simulink model "connections"  (R2020a)
settings: Solver=FixedStepAuto  StartTime=0.0  StopTime=5000  FixedStep=0.1  RelTol=1e-3
values from neighbouring files (symbols this model uses):
  east_drift_limit = 2    [wave_parameters.mat]
  k_down = 1.3    [wave_parameters.mat]
  k_east = 2    [wave_parameters.mat]
  k_north = 2    [wave_parameters.mat]
  k_pitch = 3    [wave_parameters.mat]
  k_roll = 3    [wave_parameters.mat]
  k_yaw = 3    [wave_parameters.mat]
  north_drift_limit = 2    [wave_parameters.mat]
  numberOfBuses = 2    [init.m]
  numberOfGenerators = 4    [init.m]
  peak_frequency = 0.8    [wave_parameters.mat]
  wave_height = 1    [wave_parameters.mat]
  yaw_drift_limit = 0.174532925199    [wave_parameters.mat]
undefined symbols (not defined in the file or in its folder): east, magnitude, north, surge, sway, yaw
libraries: simulink x28, simulink_extras x18
(part 3 of 4)

== system connections/power_plant/Subsystem/Bus array to array1/Bus array to array ==
  In1 : Inport  OutDataTypeStr=Bus: TheveninBus  Partition=on  PartitionDimension=2  PartitionWidth=1  PartitionOffset=0
  Bus Selector : BusSelector  OutputSignals=E,Z,Sb,Connected,omega,SwitchboardID
  For Each : ForEach  DisableCoverage=on
  E : Outport  ConcatenationDimension=2  VectorParamsAs1DForOutWhenUnconnected=off
  Z : Outport  Port=2  ConcatenationDimension=2  VectorParamsAs1DForOutWhenUnconnected=off
  Sb : Outport  Port=3  ConcatenationDimension=2  VectorParamsAs1DForOutWhenUnconnected=off
  Connected : Outport  Port=4  ConcatenationDimension=2  VectorParamsAs1DForOutWhenUnconnected=off
  omega : Outport  Port=5  ConcatenationDimension=2  VectorParamsAs1DForOutWhenUnconnected=off
  SwitchboardID : Outport  Port=6  ConcatenationDimension=2  VectorParamsAs1DForOutWhenUnconnected=off
  wires:
  Bus Selector/6 -> SwitchboardID/1  "<SwitchboardID>"
  Bus Selector/5 -> omega/1  "<omega>"
  Bus Selector/4 -> Connected/1  "<Connected>"
  Bus Selector/3 -> Sb/1  "<Sb>"
  Bus Selector/1 -> E/1  "<E>"
  Bus Selector/2 -> Z/1  "<Z>"
  In1/1 -> Bus Selector/1

== system connections/power_plant/Subsystem/Merger/For Each Subsystem ==
  v : Inport  Partition=on  PartitionDimension=2  PartitionWidth=1  PartitionOffset=0
  omega : Inport  Port=2  Partition=on  PartitionDimension=2  PartitionWidth=1  PartitionOffset=0
  theta : Inport  Port=3  Partition=on  PartitionDimension=2  PartitionWidth=1  PartitionOffset=0
  Bus Creator : BusCreator  Inputs=3  OutDataTypeStr=Bus: swb  NonVirtualBus=on
  For Each : ForEach  DisableCoverage=on
  Out1 : Outport  OutDataTypeStr=Bus: swb  ConcatenationDimension=2  VectorParamsAs1DForOutWhenUnconnected=off
  wires:
  Bus Creator/1 -> Out1/1
  v/1 -> Bus Creator/1  "voltage"
  omega/1 -> Bus Creator/2  "omega"
  theta/1 -> Bus Creator/3  "thetaElectric"

== system connections/power_plant/Subsystem1/Subsystem1/Bus array to array ==
  In1 : Inport  OutDataTypeStr=Bus: TheveninBus  Partition=on  PartitionDimension=1  PartitionWidth=1  PartitionOffset=0
  Bus array to array : Subsystem  TreatAsAtomicUnit=on
  For Each : ForEach  DisableCoverage=on
  E : Outport  ConcatenationDimension=1  VectorParamsAs1DForOutWhenUnconnected=off
  Z : Outport  Port=2  ConcatenationDimension=1  VectorParamsAs1DForOutWhenUnconnected=off
  Sb : Outport  Port=3  ConcatenationDimension=1  VectorParamsAs1DForOutWhenUnconnected=off
  Connected : Outport  Port=4  ConcatenationDimension=1  VectorParamsAs1DForOutWhenUnconnected=off
  omega : Outport  Port=5  ConcatenationDimension=1  VectorParamsAs1DForOutWhenUnconnected=off
  SwitchboardID : Outport  Port=6  ConcatenationDimension=1  VectorParamsAs1DForOutWhenUnconnected=off
  wires:
  Bus array to array/6(SwitchboardID) -> SwitchboardID/1
  Bus array to array/5(omega) -> omega/1
  Bus array to array/4(Connected) -> Connected/1
  Bus array to array/3(Sb) -> Sb/1
  Bus array to array/1(E) -> E/1
  Bus array to array/2(Z) -> Z/1
  In1/1 -> Bus array to array/1(In1)

== system connections/power_plant/Subsystem1/Subsystem1/For Each Subsystem1 ==
  E : Inport  Partition=on  PartitionDimension=1  PartitionWidth=1  PartitionOffset=0
  Z : Inport  Port=2  Partition=on  PartitionDimension=1  PartitionWidth=1  PartitionOffset=0
  Sb : Inport  Port=3  Partition=on  PartitionDimension=1  PartitionWidth=1  PartitionOffset=0
  Connected : Inport  Port=4  Partition=on  PartitionDimension=1  PartitionWidth=1  PartitionOffset=0
  omega : Inport  Port=5  Partition=on  PartitionDimension=1  PartitionWidth=1  PartitionOffset=0
  SwitchboardID : Inport  Port=6  Partition=on  PartitionDimension=1  PartitionWidth=1  PartitionOffset=0
  For Each : ForEach  DisableCoverage=on
  For Each Subsystem : Subsystem  TreatAsAtomicUnit=on
  Out1 : Outport  OutDataTypeStr=Bus: TheveninBus  ConcatenationDimension=1  VectorParamsAs1DForOutWhenUnconnected=off
  wires:
  For Each Subsystem/1(Out1) -> Out1/1
  SwitchboardID/1 -> For Each Subsystem/6(SwitchboardID)  "SwitchboardID"
  omega/1 -> For Each Subsystem/5(omega)  "omega"
  Connected/1 -> For Each Subsystem/4(Connected)  "Connected"
  Sb/1 -> For Each Subsystem/3(Sb)  "Sb"
  Z/1 -> For Each Subsystem/2(Z)  "Z"
  E/1 -> For Each Subsystem/1(E)  "E"

== system connections/power_plant/Subsystem1/Subsystem1/Logical selector to find which component is connected to this bus1 ==
  Input : Inport
  Selector : Inport  Port=2
  Relational Operator : RelationalOperator  Operator===  OutDataTypeStr=boolean  RndMeth=Simplest
  Transpose2 : Math  Operator=transpose  SignedPower=on  SaturateOnIntegerOverflow=on
  repmat : Selector  NumberOfDimensions=2  IndexOptions=Index vector (dialog),Index vector (dialog)  Indices=[1 2 3 4],ones(1,numberOfBuses)  OutputSizes=1,1
  repmat2 : Selector  NumberOfDimensions=2  IndexOptions=Index vector (dialog),Index vector (dialog)  Indices=[1 2],ones(1,numberOfGenerators)  OutputSizes=1,1
  Output : Outport  VectorParamsAs1DForOutWhenUnconnected=off
  wires:
  Transpose2/1 -> Relational Operator/2
  Relational Operator/1 -> Output/1
  Selector/1 -> repmat2/1
  repmat2/1 -> Transpose2/1
  repmat/1 -> Relational Operator/1
  Input/1 -> repmat/1

== system connections/power_plant/Subsystem1/Subsystem2/Bus array to array ==
  SwitchboardBus : Inport  OutDataTypeStr=Bus: TheveninBus  Partition=on  PartitionDimension=1  PartitionWidth=1  PartitionOffset=0
  Bus array to array2 : Subsystem  TreatAsAtomicUnit=on
  For Each : ForEach  DisableCoverage=on
  E : Outport  ConcatenationDimension=1  VectorParamsAs1DForOutWhenUnconnected=off
  Z : Outport  Port=2  ConcatenationDimension=1  VectorParamsAs1DForOutWhenUnconnected=off
  Sb : Outport  Port=3  ConcatenationDimension=1  VectorParamsAs1DForOutWhenUnconnected=off
  Connected : Outport  Port=4  ConcatenationDimension=1  VectorParamsAs1DForOutWhenUnconnected=off
  omega : Outport  Port=5  ConcatenationDimension=1  VectorParamsAs1DForOutWhenUnconnected=off
  SwitchboardID : Outport  Port=6  ConcatenationDimension=1  VectorParamsAs1DForOutWhenUnconnected=off
  wires:
  SwitchboardBus/1 -> Bus array to array2/1(SwitchboardBus)
  Bus array to array2/2(Z) -> Z/1
  Bus array to array2/1(E) -> E/1
  Bus array to array2/3(Sb) -> Sb/1
  Bus array to array2/4(Connected) -> Connected/1
  Bus array to array2/5(omega) -> omega/1
  Bus array to array2/6(SwitchboardID) -> SwitchboardID/1

== system connections/power_plant/Subsystem1/Subsystem2/Bus array to array1 ==
  SwitchboardBus : Inport  OutDataTypeStr=Bus: powerLoadsBus  Partition=on  PartitionDimension=1  PartitionWidth=1  PartitionOffset=0
  Bus array to array2 : Subsystem  TreatAsAtomicUnit=on
  For Each : ForEach  DisableCoverage=on
  p : Outport  ConcatenationDimension=1  VectorParamsAs1DForOutWhenUnconnected=off
  q : Outport  Port=2  ConcatenationDimension=1  VectorParamsAs1DForOutWhenUnconnected=off
  SwitchboardID : Outport  Port=3  ConcatenationDimension=1  VectorParamsAs1DForOutWhenUnconnected=off
  wires:
  SwitchboardBus/1 -> Bus array to array2/1(SwitchboardLoads)
  Bus array to array2/2(q) -> q/1
  Bus array to array2/1(p) -> p/1
  Bus array to array2/3(SwitchboardID) -> SwitchboardID/1

== system connections/power_plant/Subsystem1/Subsystem2/Merger ==
  v : Inport  Partition=on  PartitionDimension=1  PartitionWidth=1  PartitionOffset=0
  omega : Inport  Port=2  Partition=on  PartitionDimension=1  PartitionWidth=1  PartitionOffset=0
  theta : Inport  Port=3  Partition=on  PartitionDimension=1  PartitionWidth=1  PartitionOffset=0
  For Each : ForEach  DisableCoverage=on
  For Each Subsystem : Subsystem  TreatAsAtomicUnit=on
  Out1 : Outport  OutDataTypeStr=Bus: swb  ConcatenationDimension=1  VectorParamsAs1DForOutWhenUnconnected=off
  wires:
  For Each Subsystem/1(Out1) -> Out1/1
  v/1 -> For Each Subsystem/1(v)  "voltage"
  omega/1 -> For Each Subsystem/2(omega)  "omega"
  theta/1 -> For Each Subsystem/3(theta)  "thetaElectric"

== system connections/power_plant/Subsystem1/Subsystem2/busVoltage ==
  ET : Inport
  ZT : Inport  Port=2
  Sb_bus : Inport  Port=3
  Pbus : Inport  Port=4
  Qbus : Inport  Port=5
  Complex to Real-Imag : ComplexToRealImag
  Complex to Real-Imag1 : ComplexToRealImag
  Divide : Product  Inputs=*/
  Divide1 : Product  Inputs=*/
  For Iterator Subsystem1 : Subsystem  TreatAsAtomicUnit=on
  busVoltageIsValid : Subsystem
  v : Outport  VectorParamsAs1DForOutWhenUnconnected=off
  loadAngle : Outport  Port=2  VectorParamsAs1DForOutWhenUnconnected=off
  isInputValid : Outport  Port=3  VectorParamsAs1DForOutWhenUnconnected=off
  wires:
  Complex to Real-Imag1/1 -> busVoltageIsValid/6(zr)  "Zreal"
  Complex to Real-Imag1/2 -> busVoltageIsValid/5(zi)  "Zimag"
  Complex to Real-Imag/1 -> busVoltageIsValid/2(er)  "Ereal"
  Complex to Real-Imag/2 -> busVoltageIsValid/1(ei)  "Eimag"
  Sb_bus/1 -> Divide/2, Divide1/2
  Qbus/1 -> Divide1/1
  Pbus/1 -> Divide/1
  ZT/1 -> For Iterator Subsystem1/5(ZT), Complex to Real-Imag1/1  "ZT"
  Divide1/1 -> For Iterator Subsystem1/4(qbus), busVoltageIsValid/4(q)  "qbus"
  ET/1 -> For Iterator Subsystem1/1(ET), Complex to Real-Imag/1  "ET"
  Divide/1 -> For Iterator Subsystem1/3(pbus), busVoltageIsValid/3(p)  "pbus"
  For Iterator Subsystem1/1(v) -> v/1
  For Iterator Subsystem1/2(loadAngle) -> loadAngle/1
  For Iterator Subsystem1/3(isInputValid) -> isInputValid/1
  busVoltageIsValid/1(valid) -> For Iterator Subsystem1/2(valid)

== system connections/power_plant/Subsystem1/thrustersToBuses/Bus array to array ==
  powerLoads : Inport  OutDataTypeStr=Bus: powerLoadsBus  Partition=on  PartitionDimension=1  PartitionWidth=1  PartitionOffset=0
  Bus array to array : Subsystem  TreatAsAtomicUnit=on
  For Each : ForEach  DisableCoverage=on
  p : Outport  ConcatenationDimension=1  VectorParamsAs1DForOutWhenUnconnected=off
  q : Outport  Port=2  ConcatenationDimension=1  VectorParamsAs1DForOutWhenUnconnected=off
  SwitchboardID : Outport  Port=3  ConcatenationDimension=1  VectorParamsAs1DForOutWhenUnconnected=off
  wires:
  powerLoads/1 -> Bus array to array/1(powerLoads)
  Bus array to array/2(q) -> q/1
  Bus array to array/3(SwitchboardID) -> SwitchboardID/1
  Bus array to array/1(p) -> p/1

== system connections/power_plant/Subsystem1/thrustersToBuses/Bus array to array1 ==
  p : Inport  Partition=on  PartitionDimension=1  PartitionWidth=1  PartitionOffset=0
  q : Inport  Port=2  Partition=on  PartitionDimension=1  PartitionWidth=1  PartitionOffset=0
  SwitchboardID : Inport  Port=3  Partition=on  PartitionDimension=1  PartitionWidth=1  PartitionOffset=0
  Bus array to array1 : Subsystem  TreatAsAtomicUnit=on
  For Each : ForEach  DisableCoverage=on
  loads : Outport  ConcatenationDimension=1  VectorParamsAs1DForOutWhenUnconnected=off
  wires:
  p/1 -> Bus array to array1/1(p)  "p"
  q/1 -> Bus array to array1/2(q)  "q"
  SwitchboardID/1 -> Bus array to array1/3(SwitchboardID)  "SwitchboardID"
  Bus array to array1/1(loads) -> loads/1  "swb"

== system connections/power_plant/Subsystem1/thrustersToBuses/Logical selector to find which component is connected to this bus ==
  SwitchboardID : Inport
  Selector : Inport  Port=2
  Relational Operator : RelationalOperator  Operator===  OutDataTypeStr=boolean  RndMeth=Simplest
  Transpose : Math  Operator=transpose  SignedPower=on  SaturateOnIntegerOverflow=on
  repmat : Selector  NumberOfDimensions=2  IndexOptions=Index vector (dialog),Index vector (dialog)  Indices=-1,ones(1,numberOfBuses)  OutputSizes=1,1
  repmat1 : Selector  NumberOfDimensions=2  IndexOptions=Index vector (dialog),Index vector (dialog)  Indices=[1 2],ones(1,7)  OutputSizes=1,1
  Output : Outport  VectorParamsAs1DForOutWhenUnconnected=off
  wires:
  SwitchboardID/1 -> repmat/1
  repmat/1 -> Relational Operator/1
  Relational Operator/1 -> Output/1
  repmat1/1 -> Transpose/1
  Transpose/1 -> Relational Operator/2
  Selector/1 -> repmat1/1

== system connections/vessel_model/VesselDynamics/6DOFRotationMatrix/J1 ==
  yaw : Inport
  pitch : Inport  Port=2
  roll : Inport  Port=3
  Constant1 : Constant
  Constant2 : Constant
  Constant3 : Constant  Value=0
  Constant4 : Constant  Value=0
  Constant5 : Constant
  Constant6 : Constant  Value=0
  Gain : Gain  Gain=-1
  Gain1 : Gain  Gain=-1
  Gain2 : Gain  Gain=-1
  MatrixMultiply : Product  Inputs=3  Multiplication=Matrix(*)
  Reshape : Reshape  OutputDimensionality=Customize  OutputDimensions=[3,3]
  Reshape1 : Reshape  OutputDimensionality=Customize  OutputDimensions=[3,3]
  Reshape2 : Reshape  OutputDimensionality=Customize  OutputDimensions=[3,3]
  Selector : Selector  InputPortWidth=5  IndexOptions=Index vector (dialog)  Indices=[3 4 1 5 3 1 1 1 2]  OutputSizes=1
  Selector3 : Selector  InputPortWidth=5  IndexOptions=Index vector (dialog)  Indices=[3 1 5 1 2 1 4 1 3]  OutputSizes=1
  Selector9 : Selector  InputPortWidth=5  IndexOptions=Index vector (dialog)  Indices=[2 1 1 1 3 4 1 5 3]  OutputSizes=1
  Sin1 : Trigonometry
  Sin2 : Trigonometry
  Sin3 : Trigonometry  Operator=cos
  Sin4 : Trigonometry
  Sin5 : Trigonometry  Operator=cos
  Sin6 : Trigonometry  Operator=cos
  Vector Concatenate2 : Concatenate  NumInputs=5
  Vector Concatenate4 : Concatenate  NumInputs=5
  Vector Concatenate6 : Concatenate  NumInputs=5
  linear rotation matrix : Outport  VectorParamsAs1DForOutWhenUnconnected=off
  wires:
  pitch/1 -> Sin3/1, Sin2/1
  Constant6/1 -> Vector Concatenate6/1
  Sin3/1 -> Vector Concatenate4/3  "cYaw"
  Constant5/1 -> Vector Concatenate6/2
  MatrixMultiply/1 -> linear rotation matrix/1
  Sin1/1 -> Vector Concatenate6/4, Gain2/1  "sYaw"
  Selector/1 -> Reshape2/1
  yaw/1 -> Sin5/1, Sin4/1
  Reshape/1 -> MatrixMultiply/3
  Sin2/1 -> Gain1/1, Vector Concatenate4/4  "sYaw"
  Sin6/1 -> Vector Concatenate6/3  "cYaw"
  Sin4/1 -> Vector Concatenate2/4, Gain/1  "sYaw"
  Selector3/1 -> Reshape1/1
  Reshape1/1 -> MatrixMultiply/2
  Gain2/1 -> Vector Concatenate6/5
  Vector Concatenate6/1 -> Selector9/1
  Selector9/1 -> Reshape/1
  Gain/1 -> Vector Concatenate2/5
  Reshape2/1 -> MatrixMultiply/1
  Vector Concatenate2/1 -> Selector/1
  Vector Concatenate4/1 -> Selector3/1
  Constant1/1 -> Vector Concatenate2/2
  roll/1 -> Sin1/1, Sin6/1
  Gain1/1 -> Vector Concatenate4/5
  Constant4/1 -> Vector Concatenate4/1
  Constant2/1 -> Vector Concatenate4/2
  Constant3/1 -> Vector Concatenate2/1
  Sin5/1 -> Vector Concatenate2/3  "cYaw"

== system connections/vessel_model/VesselDynamics/6DOFRotationMatrix/J2 ==
  pitch angle : Inport
  roll angle : Inport  Port=2
  Constant : Constant  Value=[1 0 0]
  Gain3 : Gain  Gain=-1
  Reshape3 : Reshape  OutputDimensionality=Customize  OutputDimensions=[3,3]
  Sin10 : Trigonometry  Operator=cos
  Sin7 : Trigonometry
  Sin8 : Trigonometry  Operator=cos
  Sin9 : Trigonometry
  Vector Concatenate : Concatenate  NumInputs=7
  cx/cy : Product  Inputs=/*
  cxty : Product  Inputs=/**
  sx/cy : Product  Inputs=/*
  sxty : Product  Inputs=/**
  angular rotation matrix : Outport  VectorParamsAs1DForOutWhenUnconnected=off
  wires:
  Sin7/1 -> sxty/3, sx/cy/2, Gain3/1  "sx"
  pitch angle/1 -> Sin9/1, Sin10/1
  sxty/1 -> Vector Concatenate/2
  Sin9/1 -> cxty/2, sxty/2  "sy"
  roll angle/1 -> Sin7/1, Sin8/1
  cxty/1 -> Vector Concatenate/5
  Sin8/1 -> cx/cy/2, cxty/3, Vector Concatenate/3  "cx"
  sx/cy/1 -> Vector Concatenate/4
  cx/cy/1 -> Vector Concatenate/7
  Vector Concatenate/1 -> Reshape3/1
  Sin10/1 -> sx/cy/1, cx/cy/1, cxty/1, sxty/1  "cy"
  Constant/1 -> Vector Concatenate/1
  Gain3/1 -> Vector Concatenate/6
  Reshape3/1 -> angular rotation matrix/1

== system connections/wave_disturbances1/wave_response5/K_w/Sigma ==
  Hs : Inport
  A : Subsystem
  B : Subsystem
  Constant : Constant  Value=w0
  Constant2 : Constant  Value=5
  Constant5 : Constant  Value=4
  Constant6 : Constant  Value=3.3
  Divide1 : Product  Inputs=*/
  Divide3 : Product  Inputs=*/
  Divide4 : Product  Inputs=***
  Exp : Math  SaturateOnIntegerOverflow=on
  Pow : Math  Operator=pow  RndMeth=Zero  SaturateOnIntegerOverflow=on
  Sqrt : Sqrt  SaturateOnIntegerOverflow=on
  Square2 : Math  Operator=pow  SaturateOnIntegerOverflow=on
  Square4 : Math  Operator=pow  SaturateOnIntegerOverflow=on
  T1 : Subsystem
  Y : Subsystem
  sigma : Outport
  wires:
  B/1(B) -> Divide3/1
  A/1(A) -> Divide1/1
  Hs/1 -> A/1(Hs)
  Sqrt/1 -> sigma/1
  Divide4/1 -> Sqrt/1
  Pow/1 -> Divide4/3
  Y/1(Y) -> Pow/2
  Constant6/1 -> Pow/1
  Exp/1 -> Divide4/1
  Divide3/1 -> Exp/1
  Square4/1 -> Divide3/2
  Constant5/1 -> Square4/2
  Divide1/1 -> Divide4/2
  Square2/1 -> Divide1/2
  Constant2/1 -> Square2/2
  T1/1(T_1) -> A/2(T_1), B/1(T_1), Y/1(T_1)
  Constant/1 -> T1/1(w0), Square2/1, Square4/1, Y/2(w0)

== system connections/wave_disturbances1/wave_response_down/K_w/Sigma ==
  Hs : Inport
  A : Subsystem
  B : Subsystem
  Constant : Constant  Value=w0
  Constant2 : Constant  Value=5
  Constant5 : Constant  Value=4
  Constant6 : Constant  Value=3.3
  Divide1 : Product  Inputs=*/
  Divide3 : Product  Inputs=*/
  Divide4 : Product  Inputs=***
  Exp : Math  SaturateOnIntegerOverflow=on
  Pow : Math  Operator=pow  RndMeth=Zero  SaturateOnIntegerOverflow=on
  Sqrt : Sqrt  SaturateOnIntegerOverflow=on
  Square2 : Math  Operator=pow  SaturateOnIntegerOverflow=on
  Square4 : Math  Operator=pow  SaturateOnIntegerOverflow=on
  T1 : Subsystem
  Y : Subsystem
  sigma : Outport
  wires:
  Constant/1 -> Y/2(w0), Square4/1, Square2/1, T1/1(w0)
  T1/1(T_1) -> Y/1(T_1), B/1(T_1), A/2(T_1)
  Constant2/1 -> Square2/2
  Square2/1 -> Divide1/2
  Divide1/1 -> Divide4/2
  Constant5/1 -> Square4/2
  Square4/1 -> Divide3/2
  Divide3/1 -> Exp/1
  Exp/1 -> Divide4/1
  Constant6/1 -> Pow/1
  Y/1(Y) -> Pow/2
  Pow/1 -> Divide4/3
  Divide4/1 -> Sqrt/1
  Sqrt/1 -> sigma/1
  Hs/1 -> A/1(Hs)
  A/1(A) -> Divide1/1
  B/1(B) -> Divide3/1

== system connections/wave_disturbances1/wave_response_east/K_w/Sigma ==
  Hs : Inport
  A : Subsystem
  B : Subsystem
  Constant : Constant  Value=w0
  Constant2 : Constant  Value=5
  Constant5 : Constant  Value=4
  Constant6 : Constant  Value=3.3
  Divide1 : Product  Inputs=*/
  Divide3 : Product  Inputs=*/
  Divide4 : Product  Inputs=***
  Exp : Math  SaturateOnIntegerOverflow=on
  Pow : Math  Operator=pow  RndMeth=Zero  SaturateOnIntegerOverflow=on
  Sqrt : Sqrt  SaturateOnIntegerOverflow=on
  Square2 : Math  Operator=pow  SaturateOnIntegerOverflow=on
  Square4 : Math  Operator=pow  SaturateOnIntegerOverflow=on
  T1 : Subsystem
  Y : Subsystem
  sigma : Outport
  wires:
  B/1(B) -> Divide3/1
  A/1(A) -> Divide1/1
  Hs/1 -> A/1(Hs)
  Sqrt/1 -> sigma/1
  Divide4/1 -> Sqrt/1
  Pow/1 -> Divide4/3
  Y/1(Y) -> Pow/2
  Constant6/1 -> Pow/1
  Exp/1 -> Divide4/1
  Divide3/1 -> Exp/1
  Square4/1 -> Divide3/2
  Constant5/1 -> Square4/2
  Divide1/1 -> Divide4/2
  Square2/1 -> Divide1/2
  Constant2/1 -> Square2/2
  T1/1(T_1) -> A/2(T_1), B/1(T_1), Y/1(T_1)
  Constant/1 -> T1/1(w0), Square2/1, Square4/1, Y/2(w0)

== system connections/wave_disturbances1/wave_response_north/K_w/Sigma ==
  Hs : Inport
  A : Subsystem
  B : Subsystem
  Constant : Constant  Value=w0
  Constant2 : Constant  Value=5
  Constant5 : Constant  Value=4
  Constant6 : Constant  Value=3.3
  Divide1 : Product  Inputs=*/
  Divide3 : Product  Inputs=*/
  Divide4 : Product  Inputs=***
  Exp : Math  SaturateOnIntegerOverflow=on
  Pow : Math  Operator=pow  RndMeth=Zero  SaturateOnIntegerOverflow=on
  Sqrt : Sqrt  SaturateOnIntegerOverflow=on
  Square2 : Math  Operator=pow  SaturateOnIntegerOverflow=on
  Square4 : Math  Operator=pow  SaturateOnIntegerOverflow=on
  T1 : Subsystem
  Y : Subsystem
  sigma : Outport
  wires:
  Constant/1 -> Y/2(w0), Square4/1, Square2/1, T1/1(w0)
  T1/1(T_1) -> Y/1(T_1), B/1(T_1), A/2(T_1)
  Constant2/1 -> Square2/2
  Square2/1 -> Divide1/2
  Divide1/1 -> Divide4/2
  Constant5/1 -> Square4/2
  Square4/1 -> Divide3/2
  Divide3/1 -> Exp/1
  Exp/1 -> Divide4/1
  Constant6/1 -> Pow/1
  Y/1(Y) -> Pow/2
  Pow/1 -> Divide4/3
  Divide4/1 -> Sqrt/1
  Sqrt/1 -> sigma/1
  Hs/1 -> A/1(Hs)
  A/1(A) -> Divide1/1
  B/1(B) -> Divide3/1

== system connections/wave_disturbances1/wave_response_pitch/K_w/Sigma ==
  Hs : Inport
  A : Subsystem
  B : Subsystem
  Constant : Constant  Value=w0
  Constant2 : Constant  Value=5
  Constant5 : Constant  Value=4
  Constant6 : Constant  Value=3.3
  Divide1 : Product  Inputs=*/
  Divide3 : Product  Inputs=*/
  Divide4 : Product  Inputs=***
  Exp : Math  SaturateOnIntegerOverflow=on
  Pow : Math  Operator=pow  RndMeth=Zero  SaturateOnIntegerOverflow=on
  Sqrt : Sqrt  SaturateOnIntegerOverflow=on
  Square2 : Math  Operator=pow  SaturateOnIntegerOverflow=on
  Square4 : Math  Operator=pow  SaturateOnIntegerOverflow=on
  T1 : Subsystem
  Y : Subsystem
  sigma : Outport
  wires:
  Constant/1 -> Y/2(w0), Square4/1, Square2/1, T1/1(w0)
  T1/1(T_1) -> Y/1(T_1), B/1(T_1), A/2(T_1)
  Constant2/1 -> Square2/2
  Square2/1 -> Divide1/2
  Divide1/1 -> Divide4/2
  Constant5/1 -> Square4/2
  Square4/1 -> Divide3/2
  Divide3/1 -> Exp/1
  Exp/1 -> Divide4/1
  Constant6/1 -> Pow/1
  Y/1(Y) -> Pow/2
  Pow/1 -> Divide4/3
  Divide4/1 -> Sqrt/1
  Sqrt/1 -> sigma/1
  Hs/1 -> A/1(Hs)
  A/1(A) -> Divide1/1
  B/1(B) -> Divide3/1

== system connections/wave_disturbances1/wave_response_roll/K_w/Sigma ==
  Hs : Inport
  A : Subsystem
  B : Subsystem
  Constant : Constant  Value=w0
  Constant2 : Constant  Value=5
  Constant5 : Constant  Value=4
  Constant6 : Constant  Value=3.3
  Divide1 : Product  Inputs=*/
  Divide3 : Product  Inputs=*/
  Divide4 : Product  Inputs=***
  Exp : Math  SaturateOnIntegerOverflow=on
  Pow : Math  Operator=pow  RndMeth=Zero  SaturateOnIntegerOverflow=on
  Sqrt : Sqrt  SaturateOnIntegerOverflow=on
  Square2 : Math  Operator=pow  SaturateOnIntegerOverflow=on
  Square4 : Math  Operator=pow  SaturateOnIntegerOverflow=on
  T1 : Subsystem
  Y : Subsystem
  sigma : Outport
  wires:
  B/1(B) -> Divide3/1
  A/1(A) -> Divide1/1
  Hs/1 -> A/1(Hs)
  Sqrt/1 -> sigma/1
  Divide4/1 -> Sqrt/1
  Pow/1 -> Divide4/3
  Y/1(Y) -> Pow/2
  Constant6/1 -> Pow/1
  Exp/1 -> Divide4/1
  Divide3/1 -> Exp/1
  Square4/1 -> Divide3/2
  Constant5/1 -> Square4/2
  Divide1/1 -> Divide4/2
  Square2/1 -> Divide1/2
  Constant2/1 -> Square2/2
  T1/1(T_1) -> A/2(T_1), B/1(T_1), Y/1(T_1)
  Constant/1 -> T1/1(w0), Square2/1, Square4/1, Y/2(w0)

== system connections/power_plant/Subsystem1/Subsystem1/Bus array to array/Bus array to array ==
  In1 : Inport  OutDataTypeStr=Bus: TheveninBus  Partition=on  PartitionDimension=2  PartitionWidth=1  PartitionOffset=0
  Bus Selector : BusSelector  OutputSignals=E,Z,Sb,Connected,omega,SwitchboardID
  For Each : ForEach  DisableCoverage=on
  E : Outport  ConcatenationDimension=2  VectorParamsAs1DForOutWhenUnconnected=off
  Z : Outport  Port=2  ConcatenationDimension=2  VectorParamsAs1DForOutWhenUnconnected=off
  Sb : Outport  Port=3  ConcatenationDimension=2  VectorParamsAs1DForOutWhenUnconnected=off
  Connected : Outport  Port=4  ConcatenationDimension=2  VectorParamsAs1DForOutWhenUnconnected=off
  omega : Outport  Port=5  ConcatenationDimension=2  VectorParamsAs1DForOutWhenUnconnected=off
  SwitchboardID : Outport  Port=6  ConcatenationDimension=2  VectorParamsAs1DForOutWhenUnconnected=off
  wires:
  Bus Selector/6 -> SwitchboardID/1  "<SwitchboardID>"
  Bus Selector/5 -> omega/1  "<omega>"
  Bus Selector/4 -> Connected/1  "<Connected>"
  Bus Selector/3 -> Sb/1  "<Sb>"
  Bus Selector/1 -> E/1  "<E>"
  Bus Selector/2 -> Z/1  "<Z>"
  In1/1 -> Bus Selector/1

== system connections/power_plant/Subsystem1/Subsystem1/For Each Subsystem1/For Each Subsystem ==
  E : Inport  Partition=on  PartitionDimension=2  PartitionWidth=1  PartitionOffset=0
  Z : Inport  Port=2  Partition=on  PartitionDimension=2  PartitionWidth=1  PartitionOffset=0
  Sb : Inport  Port=3  Partition=on  PartitionDimension=2  PartitionWidth=1  PartitionOffset=0
  Connected : Inport  Port=4  Partition=on  PartitionDimension=2  PartitionWidth=1  PartitionOffset=0
  omega : Inport  Port=5  Partition=on  PartitionDimension=2  PartitionWidth=1  PartitionOffset=0
  SwitchboardID : Inport  Port=6  Partition=on  PartitionDimension=2  PartitionWidth=1  PartitionOffset=0
  Bus Creator : BusCreator  Inputs=6  OutDataTypeStr=Bus: TheveninBus  NonVirtualBus=on
  For Each : ForEach  DisableCoverage=on
  Out1 : Outport  OutDataTypeStr=Bus: TheveninBus  ConcatenationDimension=2  VectorParamsAs1DForOutWhenUnconnected=off
  wires:
  Bus Creator/1 -> Out1/1
  SwitchboardID/1 -> Bus Creator/6  "SwitchboardID"
  omega/1 -> Bus Creator/5  "omega"
  Connected/1 -> Bus Creator/4  "Connected"
  Sb/1 -> Bus Creator/3  "Sb"
  Z/1 -> Bus Creator/2  "Z"
  E/1 -> Bus Creator/1  "E"

== system connections/power_plant/Subsystem1/Subsystem2/Bus array to array/Bus array to array2 ==
  SwitchboardBus : Inport  OutDataTypeStr=Bus: TheveninBus  Partition=on  PartitionDimension=2  PartitionWidth=1  PartitionOffset=0
  Bus Selector : BusSelector  OutputSignals=E,Z,Sb,Connected,omega,SwitchboardID
  For Each : ForEach  DisableCoverage=on
  E : Outport  ConcatenationDimension=2  VectorParamsAs1DForOutWhenUnconnected=off
  Z : Outport  Port=2  ConcatenationDimension=2  VectorParamsAs1DForOutWhenUnconnected=off
  Sb : Outport  Port=3  ConcatenationDimension=2  VectorParamsAs1DForOutWhenUnconnected=off
  Connected : Outport  Port=4  ConcatenationDimension=2  VectorParamsAs1DForOutWhenUnconnected=off
  omega : Outport  Port=5  ConcatenationDimension=2  VectorParamsAs1DForOutWhenUnconnected=off
  SwitchboardID : Outport  Port=6  ConcatenationDimension=2  VectorParamsAs1DForOutWhenUnconnected=off
  wires:
  SwitchboardBus/1 -> Bus Selector/1
  Bus Selector/2 -> Z/1  "<Z>"
  Bus Selector/1 -> E/1  "<E>"
  Bus Selector/3 -> Sb/1  "<Sb>"
  Bus Selector/4 -> Connected/1  "<Connected>"
  Bus Selector/5 -> omega/1  "<omega>"
  Bus Selector/6 -> SwitchboardID/1  "<SwitchboardID>"

== system connections/power_plant/Subsystem1/Subsystem2/Bus array to array1/Bus array to array2 ==
  SwitchboardLoads : Inport  OutDataTypeStr=Bus: powerLoadsBus  Partition=on  PartitionDimension=2  PartitionWidth=1  PartitionOffset=0
  Bus Selector : BusSelector  OutputSignals=p,q,SwitchboardID
  For Each : ForEach  DisableCoverage=on
  p : Outport  ConcatenationDimension=2  VectorParamsAs1DForOutWhenUnconnected=off
  q : Outport  Port=2  ConcatenationDimension=2  VectorParamsAs1DForOutWhenUnconnected=off
  SwitchboardID : Outport  Port=3  ConcatenationDimension=2  VectorParamsAs1DForOutWhenUnconnected=off
  wires:
  Bus Selector/3 -> SwitchboardID/1  "<SwitchboardID>"
  Bus Selector/2 -> q/1  "<q>"
  SwitchboardLoads/1 -> Bus Selector/1
  Bus Selector/1 -> p/1  "<p>"

== system connections/power_plant/Subsystem1/Subsystem2/Merger/For Each Subsystem ==
  v : Inport  Partition=on  PartitionDimension=2  PartitionWidth=1  PartitionOffset=0
  omega : Inport  Port=2  Partition=on  PartitionDimension=2  PartitionWidth=1  PartitionOffset=0
  theta : Inport  Port=3  Partition=on  PartitionDimension=2  PartitionWidth=1  PartitionOffset=0
  Bus Creator : BusCreator  Inputs=3  OutDataTypeStr=Bus: swb  NonVirtualBus=on
  For Each : ForEach  DisableCoverage=on
  Out1 : Outport  OutDataTypeStr=Bus: swb  ConcatenationDimension=2  VectorParamsAs1DForOutWhenUnconnected=off
  wires:
  Bus Creator/1 -> Out1/1
  v/1 -> Bus Creator/1  "voltage"
  omega/1 -> Bus Creator/2  "omega"
  theta/1 -> Bus Creator/3  "thetaElectric"

== system connections/power_plant/Subsystem1/Subsystem2/busVoltage/For Iterator Subsystem1 ==
  ET : Inport
  valid : Inport  Port=2
  pbus : Inport  Port=3
  qbus : Inport  Port=4
  ZT : Inport  Port=5
  Assignment : Assignment  NumberOfDimensions=2  DiagnosticForDimensions=Warning  IndexOptions=Assign all,Index vector (port)  Indices=1,1  OutputSizes=1,1
  Assignment1 : Assignment  NumberOfDimensions=2  DiagnosticForDimensions=Warning  IndexOptions=Assign all,Index vector (port)  Indices=1,1  OutputSizes=1,1
  Assignment2 : Assignment  NumberOfDimensions=2  DiagnosticForDimensions=Warning  IndexOptions=Assign all,Index vector (port)  Indices=1,1  OutputSizes=1,1
  Constant : Constant  Value=zeros(1,numberOfBuses)
  Constant1 : Constant  Value=pi/4 * ones(1,numberOfBuses)
  Constant2 : Constant  Value=(.68+.68j) * ones(1,numberOfBuses)
  For Iterator : ForIterator  IterationLimit=numberOfBuses
  If : If  IfExpression=u1 == 0
  If Action Subsystem : Subsystem  TreatAsAtomicUnit=on
  If Action Subsystem1 : Subsystem  TreatAsAtomicUnit=on
  Merge : Merge  InitialOutput=[0+0j]
  Merge1 : Merge
  Merge2 : Merge
  Merge3 : Merge  InitialOutput=[0+0j]
  Real-Imag to Complex : RealImagToComplex
  Selector{,1..4} (5 alike) : Selector  NumberOfDimensions=2  InputPortWidth=numberOfBuses  IndexOptions=Select all,Index vector (port)  Indices=[1 3],1  OutputSizes=1,1
  Transpose : Math  Operator=transpose  SignedPower=on  SaturateOnIntegerOverflow=on
  Transpose1 : Math  Operator=transpose  SignedPower=on  SaturateOnIntegerOverflow=on
  Transpose2 : Math  Operator=transpose  SignedPower=on  SaturateOnIntegerOverflow=on
  v : Outport  VectorParamsAs1DForOutWhenUnconnected=off
  loadAngle : Outport  Port=2  VectorParamsAs1DForOutWhenUnconnected=off
  isInputValid : Outport  Port=3  VectorParamsAs1DForOutWhenUnconnected=off
  wires:
  If Action Subsystem/4(isInputValid) -> Merge2/1
  If/2 -> If Action Subsystem1/Action
  If Action Subsystem/3(loadAngle) -> Merge1/1
  If Action Subsystem1/4(isInputValid) -> Merge2/2
  If Action Subsystem1/3(loadAngle) -> Merge1/2
  If/1 -> If Action Subsystem/Action
  ET/1 -> Selector2/1
  ZT/1 -> Selector3/1
  qbus/1 -> Selector1/1
  pbus/1 -> Selector/1
  For Iterator/1 -> Selector1/2, Selector/2, Selector3/2, Selector4/2, Selector2/2, Assignment2/3, Assignment1/3, Assignment/3
  Selector1/1 -> If Action Subsystem1/4(qbus)
  Selector/1 -> If Action Subsystem1/3(pbus)
  Selector3/1 -> If Action Subsystem1/2(ZT)
  Selector2/1 -> If Action Subsystem1/1(ET)
  Assignment/1 -> v/1
  Merge2/1 -> Assignment2/2
  Merge1/1 -> Assignment1/2
  Assignment1/1 -> loadAngle/1
  Assignment2/1 -> isInputValid/1
  valid/1 -> Selector4/1
  Real-Imag to Complex/1 -> Assignment/2
  Merge/1 -> Real-Imag to Complex/2
  Merge3/1 -> Real-Imag to Complex/1
  If Action Subsystem1/1(vReal) -> Merge3/2
  If Action Subsystem/1(vReal) -> Merge3/1
  If Action Subsystem/2(vImag) -> Merge/1
  If Action Subsystem1/2(vImag) -> Merge/2
  Constant/1 -> Transpose2/1
  Constant2/1 -> Transpose/1
  Constant1/1 -> Transpose1/1
  Transpose/1 -> Assignment/1
  Transpose1/1 -> Assignment1/1
  Transpose2/1 -> Assignment2/1
  Selector4/1 -> If/1  "valid"

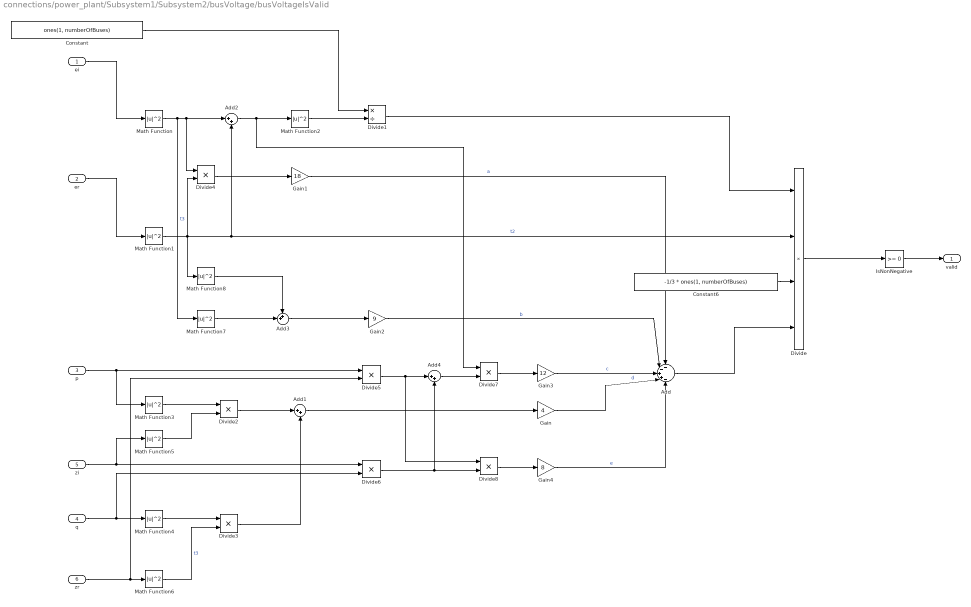
== system connections/power_plant/Subsystem1/Subsystem2/busVoltage/busVoltageIsValid ==
  ei : Inport
  er : Inport  Port=2
  p : Inport  Port=3
  q : Inport  Port=4
  zi : Inport  Port=5
  zr : Inport  Port=6
  Add : Sum  Inputs=--++-
  Add1 : Sum  Inputs=|++
  Add2 : Sum  Inputs=|++
  Add3 : Sum  Inputs=++|
  Add4 : Sum  Inputs=|++
  Constant : Constant  Value=ones(1, numberOfBuses)
  Constant6 : Constant  Value=-1/3 * ones(1, numberOfBuses)
  Divide : Product  Inputs=4
  Divide1 : Product  Inputs=*/
  Divide{2..8} (7 alike) : Product  Inputs=**
  Gain : Gain  Gain=4
  Gain1 : Gain  Gain=18
  Gain2 : Gain  Gain=9
  Gain3 : Gain  Gain=12
  Gain4 : Gain  Gain=8
  IsNonNegative : simulink/Logic and Bit Operations/Compare To Zero  relop=>=  OutDataTypeStr=boolean
  Math Function{,1..8} (9 alike) : Math  Operator=magnitude^2  SignedPower=on  SaturateOnIntegerOverflow=on
  valid : Outport  VectorParamsAs1DForOutWhenUnconnected=off
  wires:
  Math Function7/1 -> Add3/2
  Math Function8/1 -> Add3/1
  Add/1 -> Divide/4
  Gain4/1 -> Add/5  "e"
  Divide8/1 -> Gain4/1
  Gain3/1 -> Add/3  "c"
  Divide7/1 -> Gain3/1
  Add4/1 -> Divide7/2
  Gain1/1 -> Add/1  "a"
  Gain2/1 -> Add/2  "b"
  Gain/1 -> Add/4  "d"
  Divide6/1 -> Add4/2, Divide8/2
  Divide5/1 -> Add4/1, Divide8/1
  Add3/1 -> Gain2/1
  Divide4/1 -> Gain1/1
  Add1/1 -> Gain/1
  Divide3/1 -> Add1/2
  Divide2/1 -> Add1/1
  Math Function6/1 -> Divide3/2  "t3"
  Math Function4/1 -> Divide3/1
  Math Function5/1 -> Divide2/2
  Math Function3/1 -> Divide2/1
  Constant6/1 -> Divide/3
  IsNonNegative/1 -> valid/1
  zr/1 -> Math Function6/1, Divide5/2
  p/1 -> Math Function3/1, Divide5/1
  q/1 -> Divide6/2, Math Function4/1
  zi/1 -> Math Function5/1, Divide6/1
  Divide1/1 -> Divide/1
  Constant/1 -> Divide1/1
  Math Function2/1 -> Divide1/2
  Add2/1 -> Math Function2/1, Divide7/1
  Math Function/1 -> Add2/1, Divide4/1, Math Function7/1  "t3"
  Math Function1/1 -> Divide/2, Add2/2, Divide4/2, Math Function8/1  "t2"
  Divide/1 -> IsNonNegative/1
  ei/1 -> Math Function/1
  er/1 -> Math Function1/1

== system connections/power_plant/Subsystem1/thrustersToBuses/Bus array to array/Bus array to array ==
  powerLoads : Inport  OutDataTypeStr=Bus: powerLoadsBus  Partition=on  PartitionDimension=2  PartitionWidth=1  PartitionOffset=0
  Bus Selector : BusSelector  OutputSignals=p,q,SwitchboardID
  For Each : ForEach  DisableCoverage=on
  p : Outport  ConcatenationDimension=2  VectorParamsAs1DForOutWhenUnconnected=off
  q : Outport  Port=2  ConcatenationDimension=2  VectorParamsAs1DForOutWhenUnconnected=off
  SwitchboardID : Outport  Port=3  ConcatenationDimension=2  VectorParamsAs1DForOutWhenUnconnected=off
  wires:
  powerLoads/1 -> Bus Selector/1
  Bus Selector/2 -> q/1  "<q>"
  Bus Selector/3 -> SwitchboardID/1  "<SwitchboardID>"
  Bus Selector/1 -> p/1  "<p>"

== system connections/power_plant/Subsystem1/thrustersToBuses/Bus array to array1/Bus array to array1 ==
  p : Inport  Partition=on  PartitionDimension=2  PartitionWidth=1  PartitionOffset=0
  q : Inport  Port=2  Partition=on  PartitionDimension=2  PartitionWidth=1  PartitionOffset=0
  SwitchboardID : Inport  Port=3  Partition=on  PartitionDimension=2  PartitionWidth=1  PartitionOffset=0
  Bus Creator : BusCreator  Inputs=3  OutDataTypeStr=Bus: powerLoadsBus  NonVirtualBus=on
  For Each : ForEach  DisableCoverage=on
  loads : Outport  ConcatenationDimension=2  VectorParamsAs1DForOutWhenUnconnected=off
  wires:
  p/1 -> Bus Creator/1  "p"
  q/1 -> Bus Creator/2  "q"
  SwitchboardID/1 -> Bus Creator/3  "SwitchboardID"
  Bus Creator/1 -> loads/1  "swb"

== system connections/wave_disturbances1/wave_response5/K_w/Sigma/A ==
  Hs : Inport
  T_1 : Inport  Port=2
  Constant1 : Constant  Value=4
  Divide : Product  Inputs=*/
  Gain : Gain  Gain=155
  Square : Math  Operator=square  SaturateOnIntegerOverflow=on
  Square1 : Math  Operator=pow  SaturateOnIntegerOverflow=on
  A : Outport
  wires:
  T_1/1 -> Square1/1
  Divide/1 -> A/1
  Hs/1 -> Square/1
  Gain/1 -> Divide/1
  Constant1/1 -> Square1/2
  Square1/1 -> Divide/2
  Square/1 -> Gain/1

== system connections/wave_disturbances1/wave_response5/K_w/Sigma/B ==
  T_1 : Inport
  Constant3 : Constant  Value=4
  Constant4 : Constant  Value=-944
  Divide2 : Product  Inputs=*/
  Square3 : Math  Operator=pow  SaturateOnIntegerOverflow=on
  B : Outport
  wires:
  T_1/1 -> Square3/1
  Divide2/1 -> B/1
  Square3/1 -> Divide2/2
  Constant3/1 -> Square3/2
  Constant4/1 -> Divide2/1

== system connections/wave_disturbances1/wave_response5/K_w/Sigma/T1 ==
  w0 : Inport
  Constant : Constant  Value=2*pi
  Divide : Product  Inputs=*/
  Gain : Gain  Gain=0.834
  T_1 : Outport
  wires:
  Gain/1 -> T_1/1
  Divide/1 -> Gain/1
  Constant/1 -> Divide/1
  w0/1 -> Divide/2

== system connections/wave_disturbances1/wave_response5/K_w/Sigma/Y ==
  T_1 : Inport
  w0 : Inport  Port=2
  Constant : Constant
  Divide : Product  Inputs=*/
  Exp : Math  SaturateOnIntegerOverflow=on
  Gain : Gain  Gain=0.191
  Gain1 : Gain  Gain=sqrt(2)
  Gain2 : Gain  Gain=-1
  MatrixMultiply : Product
  Square : Math  Operator=square  SaturateOnIntegerOverflow=on
  Sum : Sum  Inputs=+|-
  gamma_sigma : Subsystem
  Y : Outport
  wires:
  Exp/1 -> Y/1
  Gain2/1 -> Exp/1
  Square/1 -> Gain2/1
  Divide/1 -> Square/1
  Gain1/1 -> Divide/2
  gamma_sigma/1(gamma_sigma) -> Gain1/1
  Sum/1 -> Divide/1
  Constant/1 -> Sum/2
  Gain/1 -> Sum/1
  MatrixMultiply/1 -> Gain/1
  w0/1 -> gamma_sigma/2(w0), MatrixMultiply/2
  T_1/1 -> gamma_sigma/1(T_1), MatrixMultiply/1

== system connections/wave_disturbances1/wave_response_down/K_w/Sigma/A ==
  Hs : Inport
  T_1 : Inport  Port=2
  Constant1 : Constant  Value=4
  Divide : Product  Inputs=*/
  Gain : Gain  Gain=155
  Square : Math  Operator=square  SaturateOnIntegerOverflow=on
  Square1 : Math  Operator=pow  SaturateOnIntegerOverflow=on
  A : Outport
  wires:
  Square/1 -> Gain/1
  Square1/1 -> Divide/2
  Constant1/1 -> Square1/2
  Gain/1 -> Divide/1
  Hs/1 -> Square/1
  Divide/1 -> A/1
  T_1/1 -> Square1/1

== system connections/wave_disturbances1/wave_response_down/K_w/Sigma/B ==
  T_1 : Inport
  Constant3 : Constant  Value=4
  Constant4 : Constant  Value=-944
  Divide2 : Product  Inputs=*/
  Square3 : Math  Operator=pow  SaturateOnIntegerOverflow=on
  B : Outport
  wires:
  Constant4/1 -> Divide2/1
  Constant3/1 -> Square3/2
  Square3/1 -> Divide2/2
  Divide2/1 -> B/1
  T_1/1 -> Square3/1

== system connections/wave_disturbances1/wave_response_down/K_w/Sigma/T1 ==
  w0 : Inport
  Constant : Constant  Value=2*pi
  Divide : Product  Inputs=*/
  Gain : Gain  Gain=0.834
  T_1 : Outport
  wires:
  w0/1 -> Divide/2
  Constant/1 -> Divide/1
  Divide/1 -> Gain/1
  Gain/1 -> T_1/1

== system connections/wave_disturbances1/wave_response_down/K_w/Sigma/Y ==
  T_1 : Inport
  w0 : Inport  Port=2
  Constant : Constant
  Divide : Product  Inputs=*/
  Exp : Math  SaturateOnIntegerOverflow=on
  Gain : Gain  Gain=0.191
  Gain1 : Gain  Gain=sqrt(2)
  Gain2 : Gain  Gain=-1
  MatrixMultiply : Product
  Square : Math  Operator=square  SaturateOnIntegerOverflow=on
  Sum : Sum  Inputs=+|-
  gamma_sigma : Subsystem
  Y : Outport
  wires:
  T_1/1 -> MatrixMultiply/1, gamma_sigma/1(T_1)
  w0/1 -> MatrixMultiply/2, gamma_sigma/2(w0)
  MatrixMultiply/1 -> Gain/1
  Gain/1 -> Sum/1
  Constant/1 -> Sum/2
  Sum/1 -> Divide/1
  gamma_sigma/1(gamma_sigma) -> Gain1/1
  Gain1/1 -> Divide/2
  Divide/1 -> Square/1
  Square/1 -> Gain2/1
  Gain2/1 -> Exp/1
  Exp/1 -> Y/1

== system connections/wave_disturbances1/wave_response_east/K_w/Sigma/A ==
  Hs : Inport
  T_1 : Inport  Port=2
  Constant1 : Constant  Value=4
  Divide : Product  Inputs=*/
  Gain : Gain  Gain=155
  Square : Math  Operator=square  SaturateOnIntegerOverflow=on
  Square1 : Math  Operator=pow  SaturateOnIntegerOverflow=on
  A : Outport
  wires:
  T_1/1 -> Square1/1
  Divide/1 -> A/1
  Hs/1 -> Square/1
  Gain/1 -> Divide/1
  Constant1/1 -> Square1/2
  Square1/1 -> Divide/2
  Square/1 -> Gain/1

== system connections/wave_disturbances1/wave_response_east/K_w/Sigma/B ==
  T_1 : Inport
  Constant3 : Constant  Value=4
  Constant4 : Constant  Value=-944
  Divide2 : Product  Inputs=*/
  Square3 : Math  Operator=pow  SaturateOnIntegerOverflow=on
  B : Outport
  wires:
  T_1/1 -> Square3/1
  Divide2/1 -> B/1
  Square3/1 -> Divide2/2
  Constant3/1 -> Square3/2
  Constant4/1 -> Divide2/1

== system connections/wave_disturbances1/wave_response_east/K_w/Sigma/T1 ==
  w0 : Inport
  Constant : Constant  Value=2*pi
  Divide : Product  Inputs=*/
  Gain : Gain  Gain=0.834
  T_1 : Outport
  wires:
  Gain/1 -> T_1/1
  Divide/1 -> Gain/1
  Constant/1 -> Divide/1
  w0/1 -> Divide/2

== system connections/wave_disturbances1/wave_response_east/K_w/Sigma/Y ==
  T_1 : Inport
  w0 : Inport  Port=2
  Constant : Constant
  Divide : Product  Inputs=*/
  Exp : Math  SaturateOnIntegerOverflow=on
  Gain : Gain  Gain=0.191
  Gain1 : Gain  Gain=sqrt(2)
  Gain2 : Gain  Gain=-1
  MatrixMultiply : Product
  Square : Math  Operator=square  SaturateOnIntegerOverflow=on
  Sum : Sum  Inputs=+|-
  gamma_sigma : Subsystem
  Y : Outport
  wires:
  Exp/1 -> Y/1
  Gain2/1 -> Exp/1
  Square/1 -> Gain2/1
  Divide/1 -> Square/1
  Gain1/1 -> Divide/2
  gamma_sigma/1(gamma_sigma) -> Gain1/1
  Sum/1 -> Divide/1
  Constant/1 -> Sum/2
  Gain/1 -> Sum/1
  MatrixMultiply/1 -> Gain/1
  w0/1 -> gamma_sigma/2(w0), MatrixMultiply/2
  T_1/1 -> gamma_sigma/1(T_1), MatrixMultiply/1

== system connections/wave_disturbances1/wave_response_north/K_w/Sigma/A ==
  Hs : Inport
  T_1 : Inport  Port=2
  Constant1 : Constant  Value=4
  Divide : Product  Inputs=*/
  Gain : Gain  Gain=155
  Square : Math  Operator=square  SaturateOnIntegerOverflow=on
  Square1 : Math  Operator=pow  SaturateOnIntegerOverflow=on
  A : Outport
  wires:
  Square/1 -> Gain/1
  Square1/1 -> Divide/2
  Constant1/1 -> Square1/2
  Gain/1 -> Divide/1
  Hs/1 -> Square/1
  Divide/1 -> A/1
  T_1/1 -> Square1/1

== system connections/wave_disturbances1/wave_response_north/K_w/Sigma/B ==
  T_1 : Inport
  Constant3 : Constant  Value=4
  Constant4 : Constant  Value=-944
  Divide2 : Product  Inputs=*/
  Square3 : Math  Operator=pow  SaturateOnIntegerOverflow=on
  B : Outport
  wires:
  Constant4/1 -> Divide2/1
  Constant3/1 -> Square3/2
  Square3/1 -> Divide2/2
  Divide2/1 -> B/1
  T_1/1 -> Square3/1

== system connections/wave_disturbances1/wave_response_north/K_w/Sigma/T1 ==
  w0 : Inport
  Constant : Constant  Value=2*pi
  Divide : Product  Inputs=*/
  Gain : Gain  Gain=0.834
  T_1 : Outport
  wires:
  w0/1 -> Divide/2
  Constant/1 -> Divide/1
  Divide/1 -> Gain/1
  Gain/1 -> T_1/1

== system connections/wave_disturbances1/wave_response_north/K_w/Sigma/Y ==
  T_1 : Inport
  w0 : Inport  Port=2
  Constant : Constant
  Divide : Product  Inputs=*/
  Exp : Math  SaturateOnIntegerOverflow=on
  Gain : Gain  Gain=0.191
  Gain1 : Gain  Gain=sqrt(2)
  Gain2 : Gain  Gain=-1
  MatrixMultiply : Product
  Square : Math  Operator=square  SaturateOnIntegerOverflow=on
  Sum : Sum  Inputs=+|-
  gamma_sigma : Subsystem
  Y : Outport
  wires:
  T_1/1 -> MatrixMultiply/1, gamma_sigma/1(T_1)
  w0/1 -> MatrixMultiply/2, gamma_sigma/2(w0)
  MatrixMultiply/1 -> Gain/1
  Gain/1 -> Sum/1
  Constant/1 -> Sum/2
  Sum/1 -> Divide/1
  gamma_sigma/1(gamma_sigma) -> Gain1/1
  Gain1/1 -> Divide/2
  Divide/1 -> Square/1
  Square/1 -> Gain2/1
  Gain2/1 -> Exp/1
  Exp/1 -> Y/1

== system connections/wave_disturbances1/wave_response_pitch/K_w/Sigma/A ==
  Hs : Inport
  T_1 : Inport  Port=2
  Constant1 : Constant  Value=4
  Divide : Product  Inputs=*/
  Gain : Gain  Gain=155
  Square : Math  Operator=square  SaturateOnIntegerOverflow=on
  Square1 : Math  Operator=pow  SaturateOnIntegerOverflow=on
  A : Outport
  wires:
  Square/1 -> Gain/1
  Square1/1 -> Divide/2
  Constant1/1 -> Square1/2
  Gain/1 -> Divide/1
  Hs/1 -> Square/1
  Divide/1 -> A/1
  T_1/1 -> Square1/1

== system connections/wave_disturbances1/wave_response_pitch/K_w/Sigma/B ==
  T_1 : Inport
  Constant3 : Constant  Value=4
  Constant4 : Constant  Value=-944
  Divide2 : Product  Inputs=*/
  Square3 : Math  Operator=pow  SaturateOnIntegerOverflow=on
  B : Outport
  wires:
  Constant4/1 -> Divide2/1
  Constant3/1 -> Square3/2
  Square3/1 -> Divide2/2
  Divide2/1 -> B/1
  T_1/1 -> Square3/1

== system connections/wave_disturbances1/wave_response_pitch/K_w/Sigma/T1 ==
  w0 : Inport
  Constant : Constant  Value=2*pi
  Divide : Product  Inputs=*/
  Gain : Gain  Gain=0.834
  T_1 : Outport
  wires:
  w0/1 -> Divide/2
  Constant/1 -> Divide/1
  Divide/1 -> Gain/1
  Gain/1 -> T_1/1

== system connections/wave_disturbances1/wave_response_pitch/K_w/Sigma/Y ==
  T_1 : Inport
  w0 : Inport  Port=2
  Constant : Constant
  Divide : Product  Inputs=*/
  Exp : Math  SaturateOnIntegerOverflow=on
  Gain : Gain  Gain=0.191
  Gain1 : Gain  Gain=sqrt(2)
  Gain2 : Gain  Gain=-1
  MatrixMultiply : Product
  Square : Math  Operator=square  SaturateOnIntegerOverflow=on
  Sum : Sum  Inputs=+|-
  gamma_sigma : Subsystem
  Y : Outport
  wires:
  T_1/1 -> MatrixMultiply/1, gamma_sigma/1(T_1)
  w0/1 -> MatrixMultiply/2, gamma_sigma/2(w0)
  MatrixMultiply/1 -> Gain/1
  Gain/1 -> Sum/1
  Constant/1 -> Sum/2
  Sum/1 -> Divide/1
  gamma_sigma/1(gamma_sigma) -> Gain1/1
  Gain1/1 -> Divide/2
  Divide/1 -> Square/1
  Square/1 -> Gain2/1
  Gain2/1 -> Exp/1
  Exp/1 -> Y/1

== system connections/wave_disturbances1/wave_response_roll/K_w/Sigma/A ==
  Hs : Inport
  T_1 : Inport  Port=2
  Constant1 : Constant  Value=4
  Divide : Product  Inputs=*/
  Gain : Gain  Gain=155
  Square : Math  Operator=square  SaturateOnIntegerOverflow=on
  Square1 : Math  Operator=pow  SaturateOnIntegerOverflow=on
  A : Outport
  wires:
  T_1/1 -> Square1/1
  Divide/1 -> A/1
  Hs/1 -> Square/1
  Gain/1 -> Divide/1
  Constant1/1 -> Square1/2
  Square1/1 -> Divide/2
  Square/1 -> Gain/1

== system connections/wave_disturbances1/wave_response_roll/K_w/Sigma/B ==
  T_1 : Inport
  Constant3 : Constant  Value=4
  Constant4 : Constant  Value=-944
  Divide2 : Product  Inputs=*/
  Square3 : Math  Operator=pow  SaturateOnIntegerOverflow=on
  B : Outport
  wires:
  T_1/1 -> Square3/1
  Divide2/1 -> B/1
  Square3/1 -> Divide2/2
  Constant3/1 -> Square3/2
  Constant4/1 -> Divide2/1

== system connections/wave_disturbances1/wave_response_roll/K_w/Sigma/T1 ==
  w0 : Inport
  Constant : Constant  Value=2*pi
  Divide : Product  Inputs=*/
  Gain : Gain  Gain=0.834
  T_1 : Outport
  wires:
  Gain/1 -> T_1/1
  Divide/1 -> Gain/1
  Constant/1 -> Divide/1
  w0/1 -> Divide/2

== system connections/wave_disturbances1/wave_response_roll/K_w/Sigma/Y ==
  T_1 : Inport
  w0 : Inport  Port=2
  Constant : Constant
  Divide : Product  Inputs=*/
  Exp : Math  SaturateOnIntegerOverflow=on
  Gain : Gain  Gain=0.191
  Gain1 : Gain  Gain=sqrt(2)
  Gain2 : Gain  Gain=-1
  MatrixMultiply : Product
  Square : Math  Operator=square  SaturateOnIntegerOverflow=on
  Sum : Sum  Inputs=+|-
  gamma_sigma : Subsystem
  Y : Outport
  wires:
  Exp/1 -> Y/1
  Gain2/1 -> Exp/1
  Square/1 -> Gain2/1
  Divide/1 -> Square/1
  Gain1/1 -> Divide/2
  gamma_sigma/1(gamma_sigma) -> Gain1/1
  Sum/1 -> Divide/1
  Constant/1 -> Sum/2
  Gain/1 -> Sum/1
  MatrixMultiply/1 -> Gain/1
  w0/1 -> gamma_sigma/2(w0), MatrixMultiply/2
  T_1/1 -> gamma_sigma/1(T_1), MatrixMultiply/1

== system connections/power_plant/Subsystem1/Subsystem2/busVoltage/For Iterator Subsystem1/If Action Subsystem ==
  Action Port : ActionPort  ActionPortLabel=if(u1 == 0)
  Complex to Real-Imag : ComplexToRealImag
  Constant : Constant  Value=0
  Constant1 : Constant  Value=pi/4
  Constant2 : Constant  Value=0.95
  Magnitude-Angle to Complex : MagnitudeAngleToComplex
  vReal : Outport  VectorParamsAs1DForOutWhenUnconnected=off
  vImag : Outport  Port=2  VectorParamsAs1DForOutWhenUnconnected=off
  loadAngle : Outport  Port=3  VectorParamsAs1DForOutWhenUnconnected=off
  isInputValid : Outport  Port=4  VectorParamsAs1DForOutWhenUnconnected=off
  wires:
  Constant1/1 -> loadAngle/1, Magnitude-Angle to Complex/2
  Constant2/1 -> Magnitude-Angle to Complex/1
  Constant/1 -> isInputValid/1
  Magnitude-Angle to Complex/1 -> Complex to Real-Imag/1
  Complex to Real-Imag/1 -> vReal/1
  Complex to Real-Imag/2 -> vImag/1
